simulink model "Problem3"  (R2020b)
settings: Solver=FixedStepDiscrete  StartTime=0.0  StopTime=100  RelTol=1e-3
settings Model: Creator=adity  LastModifiedBy=adity

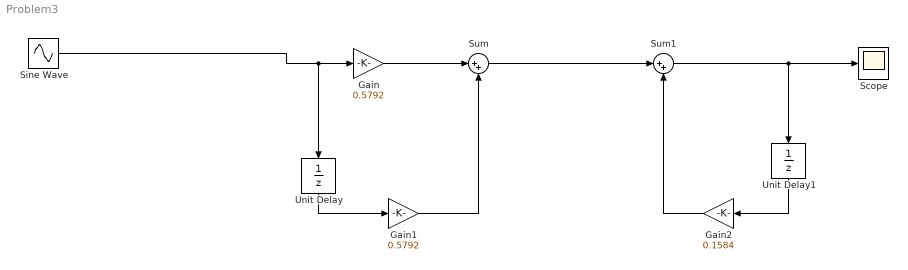
== system Problem3 ==
  Gain : Gain  Gain=0.5792
  Gain1 : Gain  Gain=0.5792
  Gain2 : Gain  Gain=0.1584
  Scope : Scope
  Sine Wave : Sin  Frequency=100  SampleTime=0
  Sum : Sum  Inputs=|++
  Sum1 : Sum  Inputs=|++
  Unit Delay : UnitDelay  SampleTime=-1  HasFrameUpgradeWarning=on
  Unit Delay1 : UnitDelay  SampleTime=-1  HasFrameUpgradeWarning=on
  wires:
  Unit Delay1/1 -> Gain2/1
  Unit Delay/1 -> Gain1/1
  Sum/1 -> Sum1/1
  Gain2/1 -> Sum1/2
  Gain/1 -> Sum/1
  Sum1/1 -> Scope/1, Unit Delay1/1
  Gain1/1 -> Sum/2
  Sine Wave/1 -> Unit Delay/1, Gain/1
